simulink model "CaseStudyII_9_Bus"  (R2020a)
settings: Solver=FixedStepAuto  StartTime=0.0  StopTime=Tend  FixedStep=T_s_power  MaxStep=5.0E-5  RelTol=1e-3
values from neighbouring files (symbols this model uses):
  B_s46 = b_s46*Cb    (= 9.5071761847e-07)    [Data_CaseStudyI.m]    (also in Data_CaseStudyII.m; Data_InitialSystem.m)
  B_s54 = b_s54*Cb    (= 1.05902722057e-06)    [Data_CaseStudyI.m]    (also in Data_CaseStudyII.m; Data_InitialSystem.m)
  B_s69 = b_s69*Cb    (= 2.15415764185e-06)    [Data_CaseStudyI.m]    (also in Data_CaseStudyII.m; Data_InitialSystem.m)
  B_s75 = b_s75*Cb    (= 1.84126323577e-06)    [Data_CaseStudyI.m]    (also in Data_CaseStudyII.m; Data_InitialSystem.m)
  B_s87 = b_s87*Cb    (= 8.96562817417e-07)    [Data_CaseStudyI.m]    (also in Data_CaseStudyII.m; Data_InitialSystem.m)
  B_s98 = b_s98*Cb    (= 1.25759482443e-06)    [Data_CaseStudyI.m]    (also in Data_CaseStudyII.m; Data_InitialSystem.m)
  C_dc_DVPP_1_2 = 0.008*(n_DVPP_1_2)    (= 0.8)    [Data_CaseStudyI.m]    (also in Data_CaseStudyII.m)
  C_dc_DVPP_1_3 = 0.008*(n_DVPP_1_3)    (= 0.4)    [Data_CaseStudyI.m]    (also in Data_CaseStudyII.m)
  C_dc_DVPP_3_1 = 0.008*(n_DVPP_3_1)    (= 1.128)    [Data_CaseStudyII.m]
  C_dc_DVPP_3_2 = 0.008*(n_DVPP_3_2)    (= 0.848)    [Data_CaseStudyII.m]
  C_dc_DVPP_3_3 = 0.008*(n_DVPP_3_3)    (= 1.28)    [Data_CaseStudyII.m]
  Dp_DVPP_3_pu = 1/dp_DVPP_3    (= 33.3333333333)    [Data_CaseStudyII.m]
  Dq1_DVPP_3_pu = 100    [Data_CaseStudyII.m]
  fb = 50    [Data_CaseStudyI.m]    (also in Data_CaseStudyII.m; Data_InitialSystem.m)
  HGov_dyn = HGov_delay*H_tr_droop    [Data_CaseStudyI.m]    (also in Data_CaseStudyII.m; Data_InitialSystem.m)
  HTurb_tot = H_water_way    [Data_CaseStudyI.m]    (also in Data_CaseStudyII.m; Data_InitialSystem.m)
  I_m_DVPP_1_2 = 2/3*Sb_DVPP_1_2/V_m_DVPP_1_2    [Data_CaseStudyI.m]    (also in Data_CaseStudyII.m)
  I_m_DVPP_1_3 = 2/3*Sb_DVPP_1_3/V_m_DVPP_1_3    [Data_CaseStudyI.m]    (also in Data_CaseStudyII.m)
  I_m_DVPP_3_1 = 2/3*Sb_DVPP_3_1/V_m_DVPP_3_1    [Data_CaseStudyII.m]
  I_m_DVPP_3_2 = 2/3*Sb_DVPP_3_2/V_m_DVPP_3_2    [Data_CaseStudyII.m]
  I_m_DVPP_3_3 = 2/3*Sb_DVPP_3_3/V_m_DVPP_3_3    [Data_CaseStudyII.m]
  i_star_max = 1.3    [Data_CaseStudyI.m]    (also in Data_CaseStudyII.m)
  iabc_DVPP_1_2_0 = T0*idq0_DVPP_1_2    [Data_CaseStudyI.m]    (also in Data_CaseStudyII.m)
  iabc_DVPP_1_3_0 = T0*idq0_DVPP_1_3    [Data_CaseStudyI.m]    (also in Data_CaseStudyII.m)
  iabc_DVPP_3_1_0 = T0*idq0_DVPP_3_1    [Data_CaseStudyII.m]
  iabc_DVPP_3_2_0 = T0*idq0_DVPP_3_2    [Data_CaseStudyII.m]
  iabc_DVPP_3_3_0 = T0*idq0_DVPP_3_3    [Data_CaseStudyII.m]
  K2_DVPP_1 = [-0.0221795494247 -1.60799665656 0.160449825826 -2.94803557381 -11.8081988371 -9.75170960256 0.00463021906909 -49.1667298155]    [ControlGains_DVPP1.mat]
  K3_DVPP_1 = [-0.0591512752956 -1.61493903379 -27.2946107927 -16.2119211358 -14.3657419818 2.05688388773 -2.27328406162 0.146700393037 -150.920793597]    [ControlGains_DVPP1.mat]
  k_dc_DVPP_1_2 = eta_DVPP_1_2/(Vdc_n_DVPP_1_2*m_p_DVPP_1_2)    [Data_CaseStudyI.m]    (also in Data_CaseStudyII.m)
  k_dc_DVPP_1_3 = eta_DVPP_1_3/(Vdc_n_DVPP_1_3*m_p_DVPP_1_3)    [Data_CaseStudyI.m]    (also in Data_CaseStudyII.m)
  k_dc_DVPP_3_1 = eta_DVPP_3_1/(Vdc_n_DVPP_3_1*m_p_DVPP_3_1)    [Data_CaseStudyII.m]
  k_dc_DVPP_3_2 = eta_DVPP_3_2/(Vdc_n_DVPP_3_2*m_p_DVPP_3_2)    [Data_CaseStudyII.m]
  k_dc_DVPP_3_3 = eta_DVPP_3_3/(Vdc_n_DVPP_3_3*m_p_DVPP_3_3)    [Data_CaseStudyII.m]
  ki_i_pu = 1.19    [Data_CaseStudyI.m]    (also in Data_CaseStudyII.m)
  ki_pll = 1700    [Data_CaseStudyI.m]    (also in Data_CaseStudyII.m)
  ki_q_pu = 0.005    [Data_CaseStudyI.m]    (also in Data_CaseStudyII.m)
  kp_i_pu = 0.73    [Data_CaseStudyI.m]    (also in Data_CaseStudyII.m)
  kp_pll = 150    [Data_CaseStudyI.m]    (also in Data_CaseStudyII.m)
  kp_q_pu = 0.05    [Data_CaseStudyI.m]    (also in Data_CaseStudyII.m)
  L1_DVPP_1_2_pu = 0.0186/m_DVPP_1_2    (= 0.000372)    [Data_CaseStudyI.m]    (also in Data_CaseStudyII.m)
  L1_DVPP_1_3_pu = 0.0186/m_DVPP_1_3    (= 0.000744)    [Data_CaseStudyI.m]    (also in Data_CaseStudyII.m)
  L1_DVPP_3_1_pu = 0.0186/m_DVPP_3_1    (= 0.000263829787234)    [Data_CaseStudyII.m]
  L1_DVPP_3_2_pu = 0.0186/m_DVPP_3_2    (= 0.000350943396226)    [Data_CaseStudyII.m]
  L1_DVPP_3_3_pu = 0.0186/m_DVPP_3_3    (= 0.0002325)    [Data_CaseStudyII.m]
  l1_MVHV1 = 0    [Data_CaseStudyI.m]    (also in Data_CaseStudyII.m; Data_InitialSystem.m)
  l1_MVHV2 = 0    [Data_CaseStudyI.m]    (also in Data_CaseStudyII.m; Data_InitialSystem.m)
  l1_MVHV3 = 0    [Data_CaseStudyI.m]    (also in Data_CaseStudyII.m; Data_InitialSystem.m)
  L2_DVPP_1_2_pu = L1_DVPP_1_2_pu    (= 0.000372)    [Data_CaseStudyI.m]    (also in Data_CaseStudyII.m)
  L2_DVPP_1_3_pu = L1_DVPP_1_3_pu    (= 0.000744)    [Data_CaseStudyI.m]    (also in Data_CaseStudyII.m)
  L2_DVPP_3_1_pu = L1_DVPP_3_1_pu    (= 0.000263829787234)    [Data_CaseStudyII.m]
  L2_DVPP_3_2_pu = L1_DVPP_3_2_pu    (= 0.000350943396226)    [Data_CaseStudyII.m]
  L2_DVPP_3_3_pu = L1_DVPP_3_3_pu    (= 0.0002325)    [Data_CaseStudyII.m]
  l2_MVHV1 = l_s14    (= 0.0576)    [Data_CaseStudyI.m]    (also in Data_CaseStudyII.m; Data_InitialSystem.m)
  l2_MVHV2 = l_s72    (= 0.0625)    [Data_CaseStudyI.m]    (also in Data_CaseStudyII.m; Data_InitialSystem.m)
  l2_MVHV3 = l_s39    (= 0.0586)    [Data_CaseStudyI.m]    (also in Data_CaseStudyII.m; Data_InitialSystem.m)
  l_f_DVPP_1_2 = L_f_DVPP_1_2*w_b/Zb_DVPP_1_2    [Data_CaseStudyI.m]    (also in Data_CaseStudyII.m)
  L_f_DVPP_1_2 = (1/(n_DVPP_1_2))*600*10^-6    (= 6e-06)    [Data_CaseStudyI.m]    (also in Data_CaseStudyII.m)
  l_f_DVPP_1_3 = L_f_DVPP_1_3*w_b/Zb_DVPP_1_3    [Data_CaseStudyI.m]    (also in Data_CaseStudyII.m)
  L_f_DVPP_1_3 = (1/(n_DVPP_1_3))*600*10^-6    (= 1.2e-05)    [Data_CaseStudyI.m]    (also in Data_CaseStudyII.m)
  l_f_DVPP_3_1 = L_f_DVPP_3_1*w_b/Zb_DVPP_3_1    [Data_CaseStudyII.m]
  L_f_DVPP_3_1 = (1/(n_DVPP_3_1))*600*10^-6    (= 4.25531914894e-06)    [Data_CaseStudyII.m]
  l_f_DVPP_3_2 = L_f_DVPP_3_2*w_b/Zb_DVPP_3_2    [Data_CaseStudyII.m]
  L_f_DVPP_3_2 = (1/(n_DVPP_3_2))*600*10^-6    (= 5.66037735849e-06)    [Data_CaseStudyII.m]
  l_f_DVPP_3_3 = L_f_DVPP_3_3*w_b/Zb_DVPP_3_3    [Data_CaseStudyII.m]
  L_f_DVPP_3_3 = (1/(n_DVPP_3_3))*600*10^-6    (= 3.75e-06)    [Data_CaseStudyII.m]
  L_s46 = l_s46*Lb    (= 0.154915055408)    [Data_CaseStudyI.m]    (also in Data_CaseStudyII.m; Data_InitialSystem.m)
  L_s54 = l_s54*Lb    (= 0.143128040323)    [Data_CaseStudyI.m]    (also in Data_CaseStudyII.m; Data_InitialSystem.m)
  L_s69 = l_s69*Lb    (= 0.286256080645)    [Data_CaseStudyI.m]    (also in Data_CaseStudyII.m; Data_InitialSystem.m)
  L_s75 = l_s75*Lb    (= 0.271101346964)    [Data_CaseStudyI.m]    (also in Data_CaseStudyII.m; Data_InitialSystem.m)
  L_s87 = l_s87*Lb    (= 0.12123786945)    [Data_CaseStudyI.m]    (also in Data_CaseStudyII.m; Data_InitialSystem.m)
  L_s98 = l_s98*Lb    (= 0.16973301723)    [Data_CaseStudyI.m]    (also in Data_CaseStudyII.m; Data_InitialSystem.m)
  LPV_K1_DVPP_3 = [0.014519129833 -1.24253756746e-17 -0.00331576987938 -1.41950397655e-17 -0.00331577010739 -1.6423216922e-19 0.0145191298795 1.47256053017e-18 1.92456501739e-17 0.00968260817745 7.5102914291e-19 0.0096826081765 ... (80 elements, 8x10)]    [ControlGains_DVPP3_LPV.mat]
  LPV_K2_DVPP_3 = [0.0299413265511 -2.72480441208e-16 -0.00563144274341 -6.63344905835e-17 -0.00563144273182 -1.08918556426e-16 0.0299413268326 -1.32404731664e-16 -4.78559537004e-17 -0.00914230292149 -8.50409089014e-21 -0.00914230292147 ... (80 elements, 8x10)]    [ControlGains_DVPP3_LPV.mat]
  LPV_K3_DVPP_3 = [-0.0173301370849 5.00398589077e-17 -0.0636125194304 3.31757376688e-17 -0.0636125164794 5.41726806116e-17 -0.017330137145 2.43427565927e-17 -0.0400570975704 -5.68753124238e-17 -0.0574012283733 2.45717741258e-17 ... (192 elements, 16x12)]    [ControlGains_DVPP3_LPV.mat]
  Mp_DVPP_3_pu = 13    [Data_CaseStudyII.m]
  P_L = pL*Sb    (= 300000000)    [Data_CaseStudyI.m]    (also in Data_CaseStudyII.m; Data_InitialSystem.m)
  p_set_bus1 = P_set_bus1/SbSG1    (= 0.731707317073)    [Data_CaseStudyI.m]    (also in Data_CaseStudyII.m; Data_InitialSystem.m)
  p_set_bus2 = P_set_bus2/SbSG2    (= 0.756707317073)    [Data_CaseStudyI.m]    (also in Data_CaseStudyII.m; Data_InitialSystem.m)
  Pb_DVPP_3_1 = 37e6    (= 37000000)    [Data_CaseStudyII.m]
  Pb_DVPP_3_2 = 28e6    (= 28000000)    [Data_CaseStudyII.m]
  Pb_DVPP_3_3 = 0e6    (= 0)    [Data_CaseStudyII.m]
  pset_DVPP_1_1 = P_set_bus1/SbSG1    (= 0.731707317073)    [Data_CaseStudyI.m]    (also in Data_CaseStudyII.m)
  pset_DVPP_1_2 = 0    [Data_CaseStudyI.m]    (also in Data_CaseStudyII.m)
  pset_DVPP_1_3 = 0    [Data_CaseStudyI.m]    (also in Data_CaseStudyII.m)
  pset_DVPP_3_1 = (0.6*P_set_bus3)/Sb_DVPP_3_1    (= 0.398546964193)    [Data_CaseStudyII.m]
  pset_DVPP_3_2 = (0.4*P_set_bus3)/Sb_DVPP_3_2    (= 0.353428439945)    [Data_CaseStudyII.m]
  pset_DVPP_3_3 = 0    [Data_CaseStudyII.m]
  Q_L = qL*Sb    (= 82500000)    [Data_CaseStudyI.m]    (also in Data_CaseStudyII.m; Data_InitialSystem.m)
  qset_DVPP_1_2 = 0    [Data_CaseStudyI.m]    (also in Data_CaseStudyII.m)
  qset_DVPP_1_3 = 0    [Data_CaseStudyI.m]    (also in Data_CaseStudyII.m)
  qset_DVPP_3_1 = 0    [Data_CaseStudyII.m]
  qset_DVPP_3_2 = 0    [Data_CaseStudyII.m]
  qset_DVPP_3_3 = 0    [Data_CaseStudyII.m]
  R1_DVPP_1_2_pu = 0.00734/m_DVPP_1_2    (= 0.0001468)    [Data_CaseStudyI.m]    (also in Data_CaseStudyII.m)
  R1_DVPP_1_3_pu = 0.00734/m_DVPP_1_3    (= 0.0002936)    [Data_CaseStudyI.m]    (also in Data_CaseStudyII.m)
  R1_DVPP_3_1_pu = 0.00734/m_DVPP_3_1    (= 0.000104113475177)    [Data_CaseStudyII.m]
  R1_DVPP_3_2_pu = 0.00734/m_DVPP_3_2    (= 0.000138490566038)    [Data_CaseStudyII.m]
  R1_DVPP_3_3_pu = 0.00734/m_DVPP_3_3    (= 9.175e-05)    [Data_CaseStudyII.m]
  r1_MVHV1 = 1e-6    (= 1e-06)    [Data_CaseStudyI.m]    (also in Data_CaseStudyII.m; Data_InitialSystem.m)
  r1_MVHV2 = 1e-6    (= 1e-06)    [Data_CaseStudyI.m]    (also in Data_CaseStudyII.m; Data_InitialSystem.m)
  r1_MVHV3 = 1e-6    (= 1e-06)    [Data_CaseStudyI.m]    (also in Data_CaseStudyII.m; Data_InitialSystem.m)
  R2_DVPP_1_2_pu = R1_DVPP_1_2_pu    (= 0.0001468)    [Data_CaseStudyI.m]    (also in Data_CaseStudyII.m)
  R2_DVPP_1_3_pu = R1_DVPP_1_3_pu    (= 0.0002936)    [Data_CaseStudyI.m]    (also in Data_CaseStudyII.m)
  R2_DVPP_3_1_pu = R1_DVPP_3_1_pu    (= 0.000104113475177)    [Data_CaseStudyII.m]
  R2_DVPP_3_2_pu = R1_DVPP_3_2_pu    (= 0.000138490566038)    [Data_CaseStudyII.m]
  R2_DVPP_3_3_pu = R1_DVPP_3_3_pu    (= 9.175e-05)    [Data_CaseStudyII.m]
  r2_MVHV1 = 1e-6    (= 1e-06)    [Data_CaseStudyI.m]    (also in Data_CaseStudyII.m; Data_InitialSystem.m)
  r2_MVHV2 = 1e-6    (= 1e-06)    [Data_CaseStudyI.m]    (also in Data_CaseStudyII.m; Data_InitialSystem.m)
  r2_MVHV3 = 1e-6    (= 1e-06)    [Data_CaseStudyI.m]    (also in Data_CaseStudyII.m; Data_InitialSystem.m)
  R_dc_DVPP_1_2 = (Vdc_n_DVPP_1_2/(0.05*(Sb_DVPP_1_2)/Vdc_n_DVPP_1_2))    [Data_CaseStudyI.m]    (also in Data_CaseStudyII.m)
  R_dc_DVPP_1_3 = (Vdc_n_DVPP_1_3/(0.05*(Sb_DVPP_1_3)/Vdc_n_DVPP_1_3))    [Data_CaseStudyI.m]    (also in Data_CaseStudyII.m)
  R_dc_DVPP_3_1 = (Vdc_n_DVPP_3_1/(0.05*(Sb_DVPP_3_1)/Vdc_n_DVPP_3_1))    [Data_CaseStudyII.m]
  R_dc_DVPP_3_2 = (Vdc_n_DVPP_3_2/(0.05*(Sb_DVPP_3_2)/Vdc_n_DVPP_3_2))    [Data_CaseStudyII.m]
  R_dc_DVPP_3_3 = (Vdc_n_DVPP_3_3/(0.05*(Sb_DVPP_3_3)/Vdc_n_DVPP_3_3))    [Data_CaseStudyII.m]
  r_f_DVPP_1_2 = R_f_DVPP_1_2/Zb_DVPP_1_2    [Data_CaseStudyI.m]    (also in Data_CaseStudyII.m)
  R_f_DVPP_1_2 = 0.02/n_DVPP_1_2    (= 0.0002)    [Data_CaseStudyI.m]    (also in Data_CaseStudyII.m)
  r_f_DVPP_1_3 = R_f_DVPP_1_3/Zb_DVPP_1_3    [Data_CaseStudyI.m]    (also in Data_CaseStudyII.m)
  R_f_DVPP_1_3 = 0.02/n_DVPP_1_3    (= 0.0004)    [Data_CaseStudyI.m]    (also in Data_CaseStudyII.m)
  r_f_DVPP_3_1 = R_f_DVPP_3_1/Zb_DVPP_3_1    [Data_CaseStudyII.m]
  ... (+104 more)
undefined symbols (not defined in the file or in its folder): A, B, C, Continuous, Dd, Efd0, gcbh, i_dc, Ka, Kf, p2set, SbSM2, sps_rtmsupport, spsST1AModel, Ta, Tb, Tb1, Tc, Tc1, Tf, VA0, VAmax, VAmin, VImax, VImin, VRmax, VRmin
libraries: powerlib x95, powerlib_meascontrol x41, cstblocks x15, sps_avr x1, simulink_extras x1, simulink x1
(part 3 of 5)

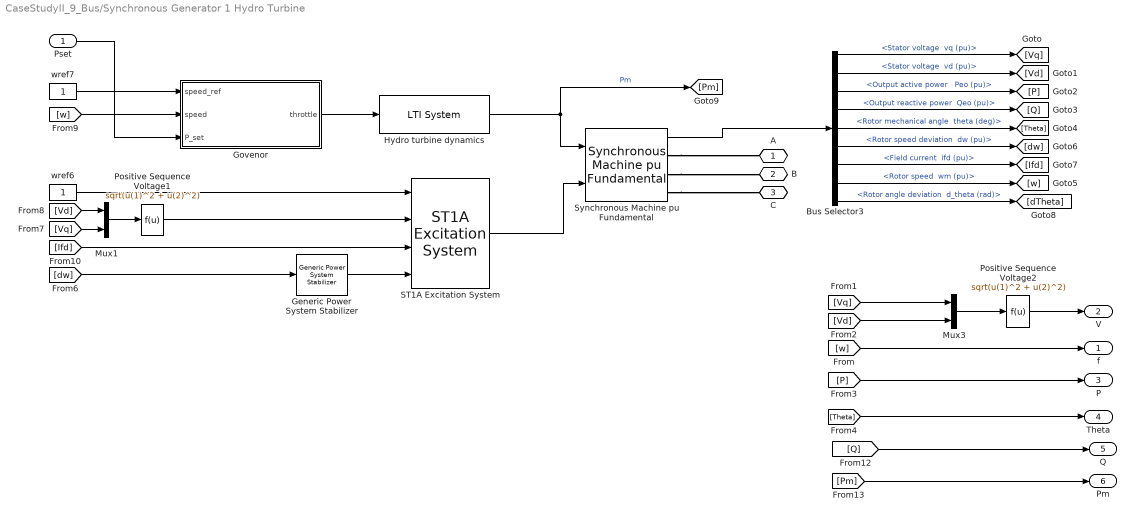
== system CaseStudyII_9_Bus/Synchronous Generator 1 Hydro Turbine ==
  Pset : Inport
  Bus Selector3 : BusSelector  OutputSignals="dq0 components.Stator voltage  vq (pu),dq0 components.Stator voltage  vd (pu),Output active power   Peo (pu),Output reactive power  Qeo (pu),Mechanical.Rotor mechanical angle  theta (deg),Mechanical.Rotor speed deviation  dw (pu),dq0 components.Field current  ifd (pu),Mechanical.Rotor speed  wm (pu),Mechanical.Rotor angle deviation  d_theta (rad)"
  Generic Power System Stabilizer : powerlib/Machines/Generic Power System Stabilizer  Tsensor=30e-3  K=15  Twashout=1  Tleadlag1=[50e-3 20e-3]  Tleadlag2=[3 5.4]  VSlimits=[-0.15 0.15]  Vinit=0  Plot_On=off  MagdB_On=on  FreqRange=logspace(-2,2,500)
      settings: SourceProductBaseCode=PS
  Govenor : Subsystem
  Hydro turbine dynamics : cstblocks/LTI System  sys=ss(HTurb_tot)  IC=p_set_bus1/3
  Mux1 : Mux  Inputs=2
  Mux3 : Mux  Inputs=2
  Positive Sequence Voltage1 : Fcn  Expr=sqrt(u(1)^2 + u(2)^2)
  Positive Sequence Voltage2 : Fcn  Expr=sqrt(u(1)^2 + u(2)^2)
  ST1A Excitation System : sps_avr/ST1A Excitation System  Tr=20e-3  KaTa=[210 0.001]  VIminmax=[-999 +999]  VAminmax=[-999 999]  VRminmax=[-6.0 6.43]  KfTf=[0.001 1]  TbTc=[0 0 0 0]  KLR=1  ILR=2  Kc=0.038  v0=[1 1.7165]  TsBlock=0
      settings: SourceProductBaseCode=PS
  Synchronous Machine pu Fundamental : powerlib/Machines/Synchronous Machine pu Fundamental  PresetModel=No  MechanicalLoad=Mechanical power Pm  ShowDetailedParameters=on  RotorType=Round  Units=per unit fundamental parameters  MeasurementBus=off  NominalParameters="[SbSG1  VbMV1   fb]"  Stator="[ 2.85E-03  0.114  1.19  0.36 ]"  Field="[ 5.79E-04  0.114]"  Dampers2=[0.0652, 0.5134, 0.0287, 0.2553, 7.765e-3, 0.9167 ]  Dampers1="[ 1.17E-02  0.182  1.97E-02  0.384 ]"  Mechanical=[6 0.0032 20]  PolePairs=20  InitialConditions=[0 0 0 0 0 0 0 0 1]  SetSaturation=off  Saturation=[0.6404,0.7127,0.8441,0.9214,0.9956,1.082,1.19,1.316,1.457;0.7,0.7698,0.8872,0.9466,0.9969,1.046,1.1,1.151,1.201]  LoadFlowParameters=[1,0,0,0,0]  TsPowergui=0  TsBlock=-1  IterativeModel=Trapezoidal non iterative  IterativeDiscreteModel=Trapezoidal non iterative  BusType=swing  Pref=p2set*SbSM2  Qref=0  Qmin=-inf  Qmax=inf  PLF=0  QLF=0
      settings: SourceProductBaseCode=PS
  wref6 : Constant
  wref7 : Constant
  A : PMIOPort  Side=Right
  B : PMIOPort  Port=2  Side=Right
  C : PMIOPort  Port=3  Side=Right
  f : Outport  VectorParamsAs1DForOutWhenUnconnected=off
  V : Outport  Port=2  VectorParamsAs1DForOutWhenUnconnected=off
  P : Outport  Port=3  VectorParamsAs1DForOutWhenUnconnected=off
  Theta : Outport  Port=4  VectorParamsAs1DForOutWhenUnconnected=off
  Q : Outport  Port=5  VectorParamsAs1DForOutWhenUnconnected=off
  Pm : Outport  Port=6  VectorParamsAs1DForOutWhenUnconnected=off
  wires:
  ST1A Excitation System/1 -> Synchronous Machine pu Fundamental/2
  [dw] -> Generic Power System Stabilizer/1
  Bus Selector3/8 -> [w]  "<Rotor speed  wm (pu)>"
  Bus Selector3/7 -> [Ifd]  "<Field current  ifd (pu)>"
  Bus Selector3/6 -> [dw]  "<Rotor speed deviation  dw (pu)>"
  Bus Selector3/5 -> [Theta]  "<Rotor mechanical angle  theta (deg)>"
  Bus Selector3/4 -> [Q]  "<Output reactive power  Qeo (pu)>"
  Bus Selector3/3 -> [P]  "<Output active power   Peo (pu)>"
  Bus Selector3/2 -> [Vd]  "<Stator voltage  vd (pu)>"
  Bus Selector3/1 -> [Vq]  "<Stator voltage  vq (pu)>"
  [Theta] -> Theta/1
  [P] -> P/1
  [Vd] -> Mux3/2
  [Vq] -> Mux3/1
  Synchronous Machine pu Fundamental/1 -> Bus Selector3/1
  Mux3/1 -> Positive Sequence Voltage2/1
  wref6/1 -> ST1A Excitation System/1
  Positive Sequence Voltage2/1 -> V/1
  [w] -> f/1
  Bus Selector3/9 -> [dTheta]  "<Rotor angle deviation  d_theta (rad)>"
  Mux1/1 -> Positive Sequence Voltage1/1
  [Vd] -> Mux1/1
  [Vq] -> Mux1/2
  Generic Power System Stabilizer/1 -> ST1A Excitation System/4
  Govenor/1(throttle) -> Hydro turbine dynamics/1
  [Q] -> Q/1
  Positive Sequence Voltage1/1 -> ST1A Excitation System/2
  [Ifd] -> ST1A Excitation System/3
  wref7/1 -> Govenor/1(speed_ref)
  Pset/1 -> Govenor/3(P_set)
  [Pm] -> Pm/1
  [w] -> Govenor/2(speed)
  Hydro turbine dynamics/1 -> Synchronous Machine pu Fundamental/1, [Pm]  "Pm"
  connections:
  Synchronous Machine pu Fundamental/RConn2 -- B/RConn1
  Synchronous Machine pu Fundamental/RConn3 -- C/RConn1
  Synchronous Machine pu Fundamental/RConn1 -- A/RConn1

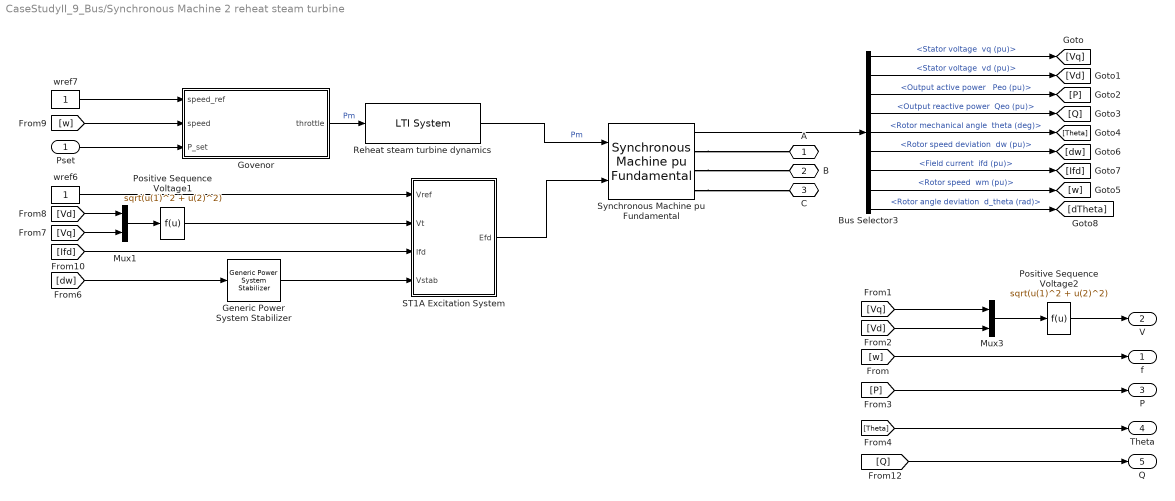
== system CaseStudyII_9_Bus/Synchronous Machine 2 reheat steam turbine ==
  Pset : Inport
  Bus Selector3 : BusSelector  OutputSignals="dq0 components.Stator voltage  vq (pu),dq0 components.Stator voltage  vd (pu),Output active power   Peo (pu),Output reactive power  Qeo (pu),Mechanical.Rotor mechanical angle  theta (deg),Mechanical.Rotor speed deviation  dw (pu),dq0 components.Field current  ifd (pu),Mechanical.Rotor speed  wm (pu),Mechanical.Rotor angle deviation  d_theta (rad)"
  Generic Power System Stabilizer : powerlib/Machines/Generic Power System Stabilizer  Tsensor=30e-3  K=15  Twashout=1  Tleadlag1=[50e-3 20e-3]  Tleadlag2=[3 5.4]  VSlimits=[-0.15 0.15]  Vinit=0  Plot_On=off  MagdB_On=on  FreqRange=logspace(-2,2,500)
      settings: SourceProductBaseCode=PS
  Govenor : Subsystem
  Mux1 : Mux  Inputs=2
  Mux3 : Mux  Inputs=2
  Positive Sequence Voltage1 : Fcn  Expr=sqrt(u(1)^2 + u(2)^2)
  Positive Sequence Voltage2 : Fcn  Expr=sqrt(u(1)^2 + u(2)^2)
  Reheat steam turbine dynamics : cstblocks/LTI System  sys=ss(STurb_reheat)  IC=[1 0.2281]
  ST1A Excitation System : Subsystem  AncestorBlock=sps_avr/ST1A Excitation System  DialogController=POWERSYS.PowerSysDialog  LoadFcn=sps_rtmsupport('LoadFcn', gcbh);  StartFcn=sps_rtmsupport('StartFcn', gcbh);  StopFcn=sps_rtmsupport('StopFcn', gcbh);  mask(ST1A Excitation System){Tr=20e-3, KaTa=[210 0.001], VIminmax=[-999 +999], VAminmax=[-999 999], VRminmax=[-6.0 6.43], KfTf=[0.001 1], TbTc=[0 0 0 0], KLR=1, ILR=2, Kc=0.038, v0=[1 1.6825], TsBlock=0}
      mask prompts: Tr "Low-pass filter time constant Tr(s):"; KaTa "Voltage regulator gain and time constant [Ka Ta(s)]:"; VIminmax "Voltage regulator input limits [VImin(pu) VImax(pu)]:"; VAminmax "Voltage regulator internal limits [VAmin(pu) VAmax(pu)]:"; VRminmax "Voltage regulator output limits [VRmin(pu) VRmax(pu)]:"; KfTf "Damping filter gain and time constant [Kf Tf(s)]:"; TbTc "Transient gain reduction lead and lag time constants [Tb(s) Tc(s) Tb1(s) Tc1(s)]:"; KLR "Exciter output current limiter gain KLR(pu):"; ILR "Exciter output current limit reference ILR(pu):"; Kc "Rectifier loading factor Kc(pu):"; v0 "Initial values of terminal voltage and field voltage [Vt0(pu) Efd0(pu)]:"; TsBlock "Sample time:"
      mask help: Implements a synchronous machine voltage regulator and exciter based on the IEEE type ST1A excitation system model. The output is the field voltage to apply to the Vf input of a Synchronous Machine block. Inputs and output are in p.u.
      mask init:
      | block = gcb;
      | [Ts,BlockChoice,MaskType,Ka,Ta,Kf,Tf,Tb,Tc,Tb1,Tc1,VRmin,VRmax,VImin,VImax,VAmin,VAmax,Ifd0,VA0,Vt0,Efd0] = powericon('ExcitationSystemInit',block,TsBlock,KaTa,KfTf,TbTc,VRminmax,VIminmax,VAminmax,Kc,ILR,KLR,v0);
      | powericon('SetInternalModels','set',block,BlockChoice);
      settings: CopyFcn=sps_rtmsupport('CopyFcn', gcbh);  DeleteFcn=sps_rtmsupport('DeleteFcn', gcbh);  UndoDeleteFcn=sps_rtmsupport('UndoDeleteFcn', gcbh);  ModelCloseFcn=sps_rtmsupport('ModelCloseFcn', gcbh);  PreSaveFcn=sps_rtmsupport('PreSaveFcn', gcbh);  PostSaveFcn=sps_rtmsupport('PostSaveFcn', gcbh);  NameChangeFcn=sps_rtmsupport('NameChangeFcn', gcbh);  PreCopyFcn=sps_rtmsupport('PreCopyFcn', gcbh);  OpenFcn=sps_rtmsupport('OpenFcn', gcbh, []);  CloseFcn=sps_rtmsupport('CloseFcn', gcbh);  PreDeleteFcn=sps_rtmsupport('PreDeleteFcn', gcbh);
      mask Help: helpview(psbhelp);
      mask Display: color('blue');disp('ST1A')
  Synchronous Machine pu Fundamental : powerlib/Machines/Synchronous Machine pu Fundamental  PresetModel=No  MechanicalLoad=Mechanical power Pm  ShowDetailedParameters=on  RotorType=Round  Units=per unit fundamental parameters  MeasurementBus=off  NominalParameters="[ SbSG2  VbMV2   fb]"  Stator="[ 2.85E-03  0.114  1.19  0.36 ]"  Field="[ 5.79E-04  0.114]"  Dampers2=[0.0652, 0.5134, 0.0287, 0.2553, 7.765e-3, 0.9167 ]  Dampers1="[ 1.17E-02  0.182  1.97E-02  0.384 ]"  Mechanical=[13 0 20]  PolePairs=20  InitialConditions=[0 0 0 0 0 0 0 0 1]  SetSaturation=off  Saturation=[0.6404,0.7127,0.8441,0.9214,0.9956,1.082,1.19,1.316,1.457;0.7,0.7698,0.8872,0.9466,0.9969,1.046,1.1,1.151,1.201]  LoadFlowParameters=[1,0,0,0,0]  TsPowergui=0  TsBlock=-1  IterativeModel=Trapezoidal non iterative  IterativeDiscreteModel=Trapezoidal non iterative  BusType=PV  Pref=P_set_bus2  Qref=0  Qmin=-inf  Qmax=inf  PLF=0  QLF=0
      settings: SourceProductBaseCode=PS
  wref6 : Constant
  wref7 : Constant
  A : PMIOPort  Side=Right
  B : PMIOPort  Port=2  Side=Right
  C : PMIOPort  Port=3  Side=Right
  f : Outport  VectorParamsAs1DForOutWhenUnconnected=off
  V : Outport  Port=2  VectorParamsAs1DForOutWhenUnconnected=off
  P : Outport  Port=3  VectorParamsAs1DForOutWhenUnconnected=off
  Theta : Outport  Port=4  VectorParamsAs1DForOutWhenUnconnected=off
  Q : Outport  Port=5  VectorParamsAs1DForOutWhenUnconnected=off
  wires:
  ST1A Excitation System/1(Efd) -> Synchronous Machine pu Fundamental/2
  [dw] -> Generic Power System Stabilizer/1
  Generic Power System Stabilizer/1 -> ST1A Excitation System/4(Vstab)
  Bus Selector3/8 -> [w]  "<Rotor speed  wm (pu)>"
  Bus Selector3/7 -> [Ifd]  "<Field current  ifd (pu)>"
  Bus Selector3/6 -> [dw]  "<Rotor speed deviation  dw (pu)>"
  Bus Selector3/5 -> [Theta]  "<Rotor mechanical angle  theta (deg)>"
  Bus Selector3/4 -> [Q]  "<Output reactive power  Qeo (pu)>"
  Bus Selector3/3 -> [P]  "<Output active power   Peo (pu)>"
  Bus Selector3/2 -> [Vd]  "<Stator voltage  vd (pu)>"
  Bus Selector3/1 -> [Vq]  "<Stator voltage  vq (pu)>"
  [Theta] -> Theta/1
  [P] -> P/1
  [Vd] -> Mux3/2
  [Vq] -> Mux3/1
  Synchronous Machine pu Fundamental/1 -> Bus Selector3/1
  Mux3/1 -> Positive Sequence Voltage2/1
  wref6/1 -> ST1A Excitation System/1(Vref)
  Positive Sequence Voltage2/1 -> V/1
  [w] -> f/1
  Bus Selector3/9 -> [dTheta]  "<Rotor angle deviation  d_theta (rad)>"
  Mux1/1 -> Positive Sequence Voltage1/1
  [Vd] -> Mux1/1
  [Vq] -> Mux1/2
  [w] -> Govenor/2(speed)
  wref7/1 -> Govenor/1(speed_ref)
  [Q] -> Q/1
  Govenor/1(throttle) -> Reheat steam turbine dynamics/1  "Pm"
  Positive Sequence Voltage1/1 -> ST1A Excitation System/2(Vt)
  [Ifd] -> ST1A Excitation System/3(Ifd)
  Pset/1 -> Govenor/3(P_set)
  Reheat steam turbine dynamics/1 -> Synchronous Machine pu Fundamental/1  "Pm"
  connections:
  Synchronous Machine pu Fundamental/RConn2 -- B/RConn1
  Synchronous Machine pu Fundamental/RConn3 -- C/RConn1
  Synchronous Machine pu Fundamental/RConn1 -- A/RConn1

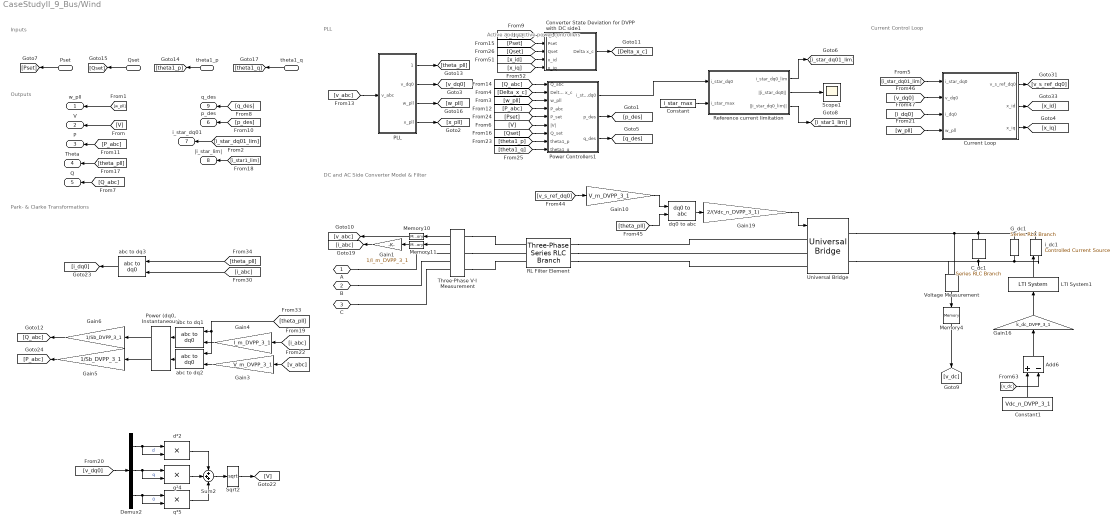
== system CaseStudyII_9_Bus/Wind  ==
  note: Current Control Loop
  note: Outputs
  note: Inputs
  note: PLL
  note: Park- & Clarke Transformations
  note: Active and reactive power controllers
  note: DC and AC Side Converter Model & Filter
  Pset : Inport
  Qset : Inport  Port=2
  theta1_p : Inport  Port=3
  theta1_q : Inport  Port=4
  Add6 : Sum  Inputs=+-
  C_dc1 : powerlib/Elements/Series RLC Branch  LConnTagsString=__new0  RConnTagsString=__new0  BranchType=C  Resistance=1  Inductance=1e-3  SetiL0=off  InitialCurrent=0  Capacitance=C_dc_DVPP_3_1  Setx0=off  InitialVoltage=Vdc_n  Measurements=None
  Constant : Constant  Value=i_star_max
  Constant1 : Constant  Value=Vdc_n_DVPP_3_1
  Converter State Deviation for DVPP with DC side1 : Subsystem
  Current Loop : Subsystem  AncestorBlock=Library/Grid-Forming Converter Controlled by Droop Control /Current Loop
  Demux2 : Demux  Outputs=3
  G_dc1 : powerlib/Elements/Series RLC Branch  LConnTagsString=__new0  RConnTagsString=__new0  BranchType=R  Resistance=R_dc_DVPP_3_1  Inductance=1e-3  SetiL0=off  InitialCurrent=0  Capacitance=1e-6  Setx0=off  InitialVoltage=0  Measurements=None
  Gain1 : Gain  Gain=1/I_m_DVPP_3_1
  Gain10 : Gain  Gain=V_m_DVPP_3_1
  Gain16 : Gain  Gain=k_dc_DVPP_3_1
  Gain19 : Gain  Gain=2/(Vdc_n_DVPP_3_1)
  Gain3 : Gain  Gain=V_m_DVPP_3_1
  Gain4 : Gain  Gain=I_m_DVPP_3_1
  Gain5 : Gain  Gain=1/Sb_DVPP_3_1
  Gain6 : Gain  Gain=1/Sb_DVPP_3_1
  LTI System1 : cstblocks/LTI System  sys=tf(1,[tau_dc_DVPP_3_1 1])  IC=[]
  Memory10 : Memory  InitialCondition=[vabc_DVPP_3_1_0_pu(1), vabc_DVPP_3_1_0_pu(2), vabc_DVPP_3_1_0_pu(3)]
  Memory11 : Memory  InitialCondition=[iabc_DVPP_3_1_0(1), iabc_DVPP_3_1_0(2), iabc_DVPP_3_1_0(3)]
  Memory4 : Memory
  PLL : Subsystem
  "Power (dq0, Instantaneous)" : powerlib_meascontrol/Measurements/Power (dq0, Instantaneous)
      settings: SourceProductBaseCode=PS
  Power Controllers1 : Subsystem
  RL Filter Element : powerlib/Elements/Three-Phase Series RLC Branch  LConnTagsString=A|B|C  RConnTagsString=A|B|C  BranchType=RL  Resistance=R_f_DVPP_3_1  Inductance=L_f_DVPP_3_1  Capacitance=0  Measurements=Branch currents
  Reference current limitation : Subsystem
  Scope1 : Scope
  Sqrt2 : Sqrt  SaturateOnIntegerOverflow=on
  Sum2 : Sum  Inputs=+++  InputSameDT=on  SaturateOnIntegerOverflow=on  OutDataTypeStr=Inherit: Same as first input
  Three-Phase V-I Measurement : powerlib/Measurements/Three-Phase V-I Measurement  VoltageMeasurement=phase-to-ground  SetLabelV=off  LabelV=Vabc  Vpu=on  VpuLL=off  CurrentMeasurement=yes  SetLabelI=off  LabelI=Iabc  Ipu=off  Pbase=Sb_conv  Vbase=VbLV_DVPP_3_1  OutputType=Complex  PhasorSimulation=off  PSBequivalent=0
  Universal Bridge : powerlib/Power Electronics/Universal Bridge  Arms=3  SnubberResistance=1e5  SnubberCapacitance=inf  Device=Average-model based VSC  Ron=1e-3  Lon=0  ForwardVoltages="[  0  0  ]"  ForwardVoltage=0  GTOparameters=[ 10e-6 , 20e-6 ]  IGBTparameters=[ 1e-6 , 2e-6 ]  Measurements=None  Measurements_2=None  converterType=Rectifier
  Voltage Measurement : powerlib/Measurements/Voltage Measurement  PhasorSimulation=off  OutputType=Complex  PSBequivalent=0
  abc to dq1 : powerlib_meascontrol/Transformations/abc to dq0  Alignment=90 degrees behind phase A axis
  abc to dq2 : powerlib_meascontrol/Transformations/abc to dq0  Alignment=90 degrees behind phase A axis
  abc to dq3 : powerlib_meascontrol/Transformations/abc to dq0  Alignment=90 degrees behind phase A axis
  dq0 to abc : powerlib_meascontrol/Transformations/dq0 to abc  Alignment=90 degrees behind phase A axis
  d²2 : Product  InputSameDT=on  RndMeth=Zero  SaturateOnIntegerOverflow=on  OutDataTypeStr=Inherit: Same as first input
  i_dc1 : powerlib/Electrical Sources/Controlled Current Source  Initialize=off  Source_Type=DC  Amplitude=i_dc  Phase=0  Frequency=0  Measurements=None
  q²4 : Product  InputSameDT=on  RndMeth=Zero  SaturateOnIntegerOverflow=on  OutDataTypeStr=Inherit: Same as first input
  q²5 : Product  InputSameDT=on  RndMeth=Zero  SaturateOnIntegerOverflow=on  OutDataTypeStr=Inherit: Same as first input
  A : PMIOPort  Side=Right
  B : PMIOPort  Port=2  Side=Right
  C : PMIOPort  Port=3  Side=Right
  w_pll : Outport  VectorParamsAs1DForOutWhenUnconnected=off
  V : Outport  Port=2  VectorParamsAs1DForOutWhenUnconnected=off
  P : Outport  Port=3  VectorParamsAs1DForOutWhenUnconnected=off
  Theta : Outport  Port=4  VectorParamsAs1DForOutWhenUnconnected=off
  Q : Outport  Port=5  VectorParamsAs1DForOutWhenUnconnected=off
  p_des : Outport  Port=6  VectorParamsAs1DForOutWhenUnconnected=off
  i_star_dq01 : Outport  Port=7  VectorParamsAs1DForOutWhenUnconnected=off
  |i_star_lim| : Outport  Port=8  VectorParamsAs1DForOutWhenUnconnected=off
  q_des : Outport  Port=9  VectorParamsAs1DForOutWhenUnconnected=off
  wires:
  Memory11/1 -> Gain1/1
  [theta_pll] -> Theta/1
  [P_abc] -> P/1
  Voltage Measurement/1 -> Memory4/1
  Three-Phase V-I Measurement/1 -> Memory10/1
  [v_dq0] -> Demux2/1
  Reference current limitation/3(||i_star_dq0_lim||) -> [i_star1_lim]
  [v_s_ref_dq0] -> Gain10/1
  Memory4/1 -> [v_dc]
  Current Loop/1(v_s_ref_dq0) -> [v_s_ref_dq0]
  Constant1/1 -> Add6/1
  abc to dq3/1 -> [i_dq0]
  [theta_pll] -> abc to dq3/2
  Demux2/2 -> q²4/1, q²4/2  "q"
  [w_pll] -> Current Loop/4(w_pll)
  Reference current limitation/1(i_star_dq0_lim) -> [i_star_dq01_lim]
  Gain16/1 -> LTI System1/1
  [theta_pll] -> dq0 to abc/2
  Gain19/1 -> Universal Bridge/1
  [v_abc] -> PLL/1(v_abc)
  [theta_pll] -> abc to dq2/2, abc to dq1/2
  Sqrt2/1 -> [V]
  "Power (dq0, Instantaneous)"/1 -> Gain5/1
  [i_abc] -> abc to dq3/1
  abc to dq2/1 -> "Power (dq0, Instantaneous)"/1
  [Q_abc] -> Q/1
  "Power (dq0, Instantaneous)"/2 -> Gain6/1
  [v_dc] -> Add6/2
  q²5/1 -> Sum2/3
  Add6/1 -> Gain16/1
  dq0 to abc/1 -> Gain19/1
  [i_star1_lim] -> |i_star_lim|/1
  Demux2/3 -> q²5/2, q²5/1  "0"
  Gain6/1 -> [Q_abc]
  Gain5/1 -> [P_abc]
  Sum2/1 -> Sqrt2/1
  Gain10/1 -> dq0 to abc/1
  [i_star_dq01_lim] -> i_star_dq01/1
  d²2/1 -> Sum2/1
  PLL/1(theta_pll) -> [theta_pll]
  [i_dq0] -> Current Loop/3(i_dq0)
  Gain1/1 -> [i_abc]
  [i_abc] -> Gain4/1
  [v_abc] -> Gain3/1
  [w_pll] -> w_pll/1
  Current Loop/2(x_id) -> [x_id]
  [V] -> V/1
  [v_dq0] -> Current Loop/2(v_dq0)
  Pset/1 -> [Pset]
  Qset/1 -> [Qset]
  Three-Phase V-I Measurement/2 -> Memory11/1
  Constant/1 -> Reference current limitation/2(i_star_max)
  abc to dq1/1 -> "Power (dq0, Instantaneous)"/2
  Gain3/1 -> abc to dq2/1
  PLL/3(w_pll) -> [w_pll]
  Reference current limitation/2(||i_star_dq0||) -> Scope1/1
  Demux2/1 -> d²2/1, d²2/2  "d"
  Memory10/1 -> [v_abc]
  Gain4/1 -> abc to dq1/1
  [p_des] -> p_des/1
  Power Controllers1/2(p_des) -> [p_des]
  PLL/2(v_dq0) -> [v_dq0]
  PLL/4(x_pll) -> [x_pll]
  q²4/1 -> Sum2/2
  Current Loop/3(x_iq) -> [x_iq]
  Power Controllers1/3(q_des) -> [q_des]
  [V] -> Power Controllers1/6(|V|)
  [Pset] -> Power Controllers1/5(P_set)
  [P_abc] -> Power Controllers1/4(P_abc)
  [w_pll] -> Power Controllers1/3(w_pll)
  [Delta_x_c] -> Power Controllers1/2(Delta x_c)
  [Q_abc] -> Power Controllers1/1(Q_abc)
  [q_des] -> q_des/1
  [Qset] -> Converter State Deviation for DVPP with DC side1/3(Qset)
  [i_dq0] -> Converter State Deviation for DVPP with DC side1/1(i_dq0)
  [x_id] -> Converter State Deviation for DVPP with DC side1/4(x_id)
  Converter State Deviation for DVPP with DC side1/1(Delta x_c) -> [Delta_x_c]
  [Pset] -> Converter State Deviation for DVPP with DC side1/2(Pset)
  [x_iq] -> Converter State Deviation for DVPP with DC side1/5(x_iq)
  [Qset] -> Power Controllers1/7(Q_set)
  theta1_p/1 -> [theta1_p]
  theta1_q/1 -> [theta1_q]
  [theta1_p] -> Power Controllers1/8(theta1_p)
  [theta1_q] -> Power Controllers1/9(theta1_q)
  LTI System1/1 -> i_dc1/1
  Power Controllers1/1(i_star_dq0) -> Reference current limitation/1(i_star_dq0)
  [i_star_dq01_lim] -> Current Loop/1(i_star_dq0)
  connections:
  Universal Bridge/RConn1 -- C_dc1/LConn1 -- i_dc1/RConn1 -- G_dc1/LConn1 -- Voltage Measurement/LConn1
  Voltage Measurement/LConn2 -- Universal Bridge/RConn2 -- C_dc1/RConn1 -- i_dc1/LConn1 -- G_dc1/RConn1
  A/RConn1 -- Three-Phase V-I Measurement/RConn1
  RL Filter Element/RConn2 -- Universal Bridge/LConn2
  B/RConn1 -- Three-Phase V-I Measurement/RConn2
  C/RConn1 -- Three-Phase V-I Measurement/RConn3
  RL Filter Element/RConn3 -- Universal Bridge/LConn3
  Three-Phase V-I Measurement/LConn2 -- RL Filter Element/LConn2
  RL Filter Element/RConn1 -- Universal Bridge/LConn1
  Three-Phase V-I Measurement/LConn1 -- RL Filter Element/LConn1
  Three-Phase V-I Measurement/LConn3 -- RL Filter Element/LConn3

== system CaseStudyII_9_Bus/BESS/Converter State Deviation ==
  i_dq0 : Inport
  x_id : Inport  Port=2
  pset : Inport  Port=3
  Constant1 : Constant  Value=xid0_DVPP_1_2_pu
  Demux2 : Demux  Outputs=3
  Gain : Gain  Gain=1/vd0_DVPP_1_2_pu
  Mux : Mux  Inputs=2
  Sum : Sum  Inputs=-+|
  Sum1 : Sum  Inputs=|+-
  Delta x_c : Outport
  wires:
  i_dq0/1 -> Demux2/1
  pset/1 -> Gain/1
  Sum/1 -> Mux/1
  Demux2/1 -> Sum/2
  Gain/1 -> Sum/1
  x_id/1 -> Sum1/1
  Constant1/1 -> Sum1/2
  Mux/1 -> Delta x_c/1
  Sum1/1 -> Mux/2

== system CaseStudyII_9_Bus/BESS/Current Loop ==
  i_star_dq0 : Inport
  v_dq0 : Inport  Port=2
  i_dq0 : Inport  Port=3
  w_pll : Inport  Port=4
  Demux : Demux  Outputs=2
  Demux1 : Demux  Outputs=2
  Demux2 : Demux  Outputs=2
  Gain : Gain  Gain=kp_i_pu
  Gain1 : Gain  Gain=ki_i_pu
  Gain2 : Gain  Gain=kp_i_pu
  Gain3 : Gain  Gain=ki_i_pu
  Gain4 : Gain  Gain=w_b
  Integrator1 : Integrator  InitialCondition=xid0_DVPP_1_2_pu
  Integrator2 : Integrator  InitialCondition=xiq0_DVPP_1_2_pu
  Memory2 : Memory
  Mux : Mux  Inputs=3
  Product : Product
  Product1 : Product
  Rf : Gain  Gain=r_f_DVPP_1_2
  Rf1 : Gain  Gain=r_f_DVPP_1_2
  Selector1 : Selector  InputPortWidth=3  IndexOptions=Index vector (dialog)  Indices=[1 2]  OutputSizes=1
  Selector2 : Selector  InputPortWidth=3  IndexOptions=Index vector (dialog)  Indices=[1 2]  OutputSizes=1
  Selector3 : Selector  InputPortWidth=3  IndexOptions=Index vector (dialog)  Indices=[1 2]  OutputSizes=1
  Sum : Sum  Inputs=|+-
  Sum1 : Sum
  Sum2 : Sum  Inputs=|+-+
  Sum3 : Sum  Inputs=|++
  Sum4 : Sum
  Sum5 : Sum  Inputs=+++|
  Sum6 : Sum  Inputs=-+|
  Sum7 : Sum  Inputs=++|
  vs_0* : Constant  Value=0
  w*Lf : Gain  Gain=l_f_DVPP_1_2/w_b
  w*Lf1 : Gain  Gain=l_f_DVPP_1_2/w_b
  v_s_ref_dq0 : Outport  VectorParamsAs1DForOutWhenUnconnected=off
  x_id : Outport  Port=2  VectorParamsAs1DForOutWhenUnconnected=off
  wires:
  vs_0*/1 -> Mux/3
  Selector3/1 -> Demux2/1
  i_dq0/1 -> Selector2/1
  Selector2/1 -> Demux1/1
  Mux/1 -> v_s_ref_dq0/1
  Sum2/1 -> Sum3/1
  v_dq0/1 -> Selector3/1
  i_star_dq0/1 -> Selector1/1
  w*Lf/1 -> Sum2/2
  Sum7/1 -> Mux/2  "vs_q*"
  Sum3/1 -> Mux/1  "vs_d*"
  Sum5/1 -> Sum7/2
  Rf/1 -> Sum2/3
  Rf1/1 -> Sum5/3
  Sum/1 -> Integrator1/1, Gain/1
  Sum1/1 -> Sum2/1
  Selector1/1 -> Demux/1
  Demux/2 -> Sum6/2
  Demux/1 -> Sum/1
  w*Lf1/1 -> Sum5/1
  Demux2/1 -> Sum3/2
  Demux2/2 -> Sum7/1
  Demux1/1 -> Product/1, Rf/1, Sum/2
  Demux1/2 -> Product1/1, Rf1/1, Sum6/1
  Gain/1 -> Sum1/1
  Gain1/1 -> Sum1/2
  Gain2/1 -> Sum4/1
  Sum6/1 -> Integrator2/1, Gain2/1
  Sum4/1 -> Sum5/2
  Gain3/1 -> Sum4/2
  Integrator2/1 -> Gain3/1
  Integrator1/1 -> Memory2/1, Gain1/1
  w_pll/1 -> Gain4/1
  Product/1 -> w*Lf1/1
  Product1/1 -> w*Lf/1
  Gain4/1 -> Product1/2, Product/2
  Memory2/1 -> x_id/1

== system CaseStudyII_9_Bus/BESS/PLL ==
  v_abc : Inport
  Display : Display
  Gain : Gain  Gain=1/fb
  Integrator3 : Integrator  InitialCondition=xpll0_pu
  Selector : Selector  InputPortWidth=3  IndexOptions=Index vector (dialog)  Indices=2  OutputSizes=1
  Subsystem : Subsystem
  abc to dq0 : powerlib_meascontrol/Transformations/abc to dq0  Alignment=90 degrees behind phase A axis
  theta_pll : Outport  VectorParamsAs1DForOutWhenUnconnected=off
  v_dq0 : Outport  Port=2  VectorParamsAs1DForOutWhenUnconnected=off
  w_pll : Outport  Port=3  VectorParamsAs1DForOutWhenUnconnected=off
  x_pll : Outport  Port=4  VectorParamsAs1DForOutWhenUnconnected=off
  wires:
  Gain/1 -> w_pll/1
  Integrator3/1 -> x_pll/1
  v_abc/1 -> Subsystem/1(Vabc), abc to dq0/1
  abc to dq0/1 -> Selector/1, v_dq0/1
  Subsystem/1(Freq) -> Display/1, Gain/1
  Subsystem/2(wt) -> abc to dq0/2, theta_pll/1
  Selector/1 -> Integrator3/1

== system CaseStudyII_9_Bus/BESS/Power Controllers ==
  Q_abc : Inport
  P_abc : Inport  Port=2
  Q_set : Inport  Port=3
  Delta x_c : Inport  Port=4
  w_pll : Inport  Port=5
  P_set : Inport  Port=6
  0 : Constant  Value=0
  DVPP State Feedback Controller for Active Power Control : Subsystem
  Mux : Mux  Inputs=3
  Reactive Power Controller PI-droop control : Subsystem
  i_star_dq0 : Outport
  p_des : Outport  Port=2
  wires:
  Mux/1 -> i_star_dq0/1
  0/1 -> Mux/3
  DVPP State Feedback Controller for Active Power Control/1(p_des) -> p_des/1
  w_pll/1 -> DVPP State Feedback Controller for Active Power Control/3(w_pll)
  P_abc/1 -> DVPP State Feedback Controller for Active Power Control/1(P_abc)
  Reactive Power Controller PI-droop control/1(i_star_q) -> Mux/2
  Q_abc/1 -> Reactive Power Controller PI-droop control/1(Q_abc)
  Q_set/1 -> Reactive Power Controller PI-droop control/2(Qset)
  Delta x_c/1 -> DVPP State Feedback Controller for Active Power Control/2(Delta_x_c)
  DVPP State Feedback Controller for Active Power Control/2(i_star_d) -> Mux/1
  P_set/1 -> DVPP State Feedback Controller for Active Power Control/4(Pset)

== system CaseStudyII_9_Bus/BESS/Reference current limitation ==
  i_star_dq0 : Inport
  i_star_max : Inport  Port=2
  Demux1 : Demux  Outputs=3
  Demux2 : Demux  Outputs=3
  Divide : Product  Inputs=*/
  Minus : Sum  Inputs=+-
  Minus1 : Sum  Inputs=+++
  Minus4 : Sum  Inputs=+++
  Product{,1..4,6..7} (7 alike) : Product  RndMeth=Zero
  Saturation1 : Saturate  UpperLimit=inf  LowerLimit=0
  Sign : Signum
  Sqrt1 : Sqrt  SaturateOnIntegerOverflow=on
  Sqrt2 : Sqrt  SaturateOnIntegerOverflow=on
  Switch1 : Switch  Threshold=1
  i_star_dq0_lim : Outport  VectorParamsAs1DForOutWhenUnconnected=off
  ||i_star_dq0|| : Outport  Port=2  VectorParamsAs1DForOutWhenUnconnected=off
  ||i_star_dq0_lim|| : Outport  Port=3  VectorParamsAs1DForOutWhenUnconnected=off
  wires:
  Sqrt2/1 -> ||i_star_dq0_lim||/1
  Minus1/1 -> Sqrt2/1
  Demux2/2 -> Product3/2, Product3/1
  Product3/1 -> Minus1/2
  Demux2/1 -> Product2/1, Product2/2
  Product4/1 -> Minus1/3
  Demux2/3 -> Product4/2, Product4/1
  Product2/1 -> Minus1/1
  i_star_max/1 -> Product6/2, Minus/2
  i_star_dq0/1 -> Switch1/3, Demux1/1, Divide/1
  Switch1/1 -> i_star_dq0_lim/1, Demux2/1
  Demux1/3 -> Product7/2, Product7/1
  Product7/1 -> Minus4/3
  Product6/1 -> Switch1/1
  Divide/1 -> Product6/1
  Sign/1 -> Switch1/2
  Saturation1/1 -> Sign/1
  Demux1/2 -> Product1/2, Product1/1
  Product/1 -> Minus4/1
  Product1/1 -> Minus4/2
  Demux1/1 -> Product/1, Product/2
  Minus4/1 -> Sqrt1/1
  Sqrt1/1 -> Minus/1, ||i_star_dq0||/1, Divide/2
  Minus/1 -> Saturation1/1

== system CaseStudyII_9_Bus/PV/Converter State Deviation for DVPP with DC side ==
  i_dq0 : Inport
  Pset : Inport  Port=2
  Qset : Inport  Port=3
  x_id : Inport  Port=4
  x_iq : Inport  Port=5
  Demux2 : Demux  Outputs=3
  Gain : Gain  Gain=1/vd0_DVPP_3_2_pu
  Gain1 : Gain  Gain=-1/vd0_DVPP_3_2_pu
  Mux : Mux
  Sum1 : Sum  Inputs=+-
  Sum2 : Sum  Inputs=-+
  Sum3 : Sum  Inputs=+-
  Sum4 : Sum  Inputs=+-
  x_id_2_pu : Constant  Value=xid0_DVPP_3_2_pu
  x_iq_2_pu : Constant  Value=xiq0_DVPP_3_2_pu
  Delta x_c : Outport
  wires:
  i_dq0/1 -> Demux2/1
  Demux2/1 -> Sum2/2
  Demux2/2 -> Sum1/1
  Sum2/1 -> Mux/1
  Sum1/1 -> Mux/2
  Gain1/1 -> Sum1/2
  Pset/1 -> Gain/1
  Gain/1 -> Sum2/1
  Qset/1 -> Gain1/1
  x_id/1 -> Sum3/1
  Sum3/1 -> Mux/3
  x_id_2_pu/1 -> Sum3/2
  Mux/1 -> Delta x_c/1
  Sum4/1 -> Mux/4
  x_iq_2_pu/1 -> Sum4/2
  x_iq/1 -> Sum4/1

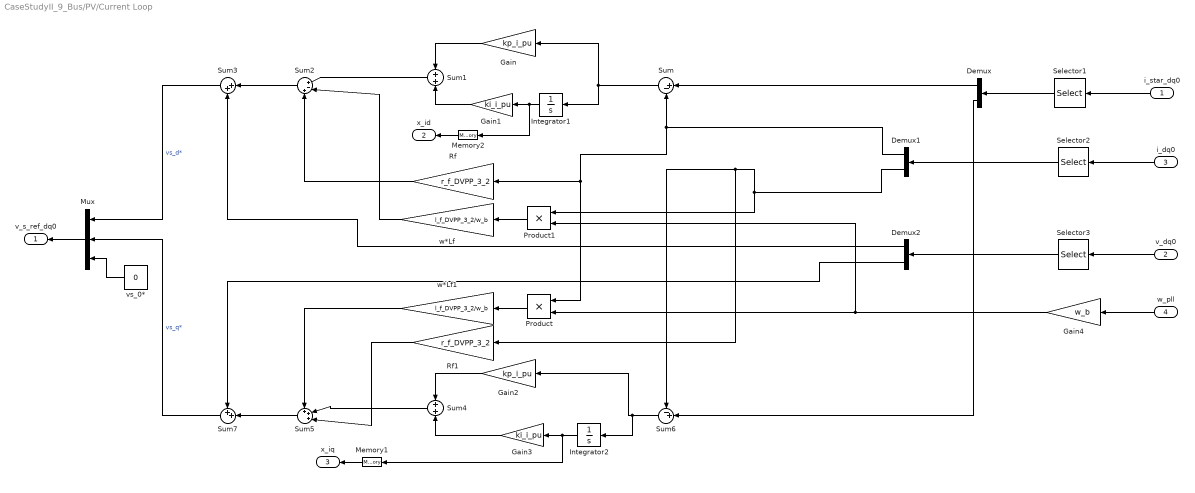
== system CaseStudyII_9_Bus/PV/Current Loop ==
  i_star_dq0 : Inport
  v_dq0 : Inport  Port=2
  i_dq0 : Inport  Port=3
  w_pll : Inport  Port=4
  Demux : Demux  Outputs=2
  Demux1 : Demux  Outputs=2
  Demux2 : Demux  Outputs=2
  Gain : Gain  Gain=kp_i_pu
  Gain1 : Gain  Gain=ki_i_pu
  Gain2 : Gain  Gain=kp_i_pu
  Gain3 : Gain  Gain=ki_i_pu
  Gain4 : Gain  Gain=w_b
  Integrator1 : Integrator  InitialCondition=xid0_DVPP_3_2_pu
  Integrator2 : Integrator  InitialCondition=xiq0_DVPP_3_2_pu
  Memory1 : Memory
  Memory2 : Memory
  Mux : Mux  Inputs=3
  Product : Product
  Product1 : Product
  Rf : Gain  Gain=r_f_DVPP_3_2
  Rf1 : Gain  Gain=r_f_DVPP_3_2
  Selector1 : Selector  InputPortWidth=3  IndexOptions=Index vector (dialog)  Indices=[1 2]  OutputSizes=1
  Selector2 : Selector  InputPortWidth=3  IndexOptions=Index vector (dialog)  Indices=[1 2]  OutputSizes=1
  Selector3 : Selector  InputPortWidth=3  IndexOptions=Index vector (dialog)  Indices=[1 2]  OutputSizes=1
  Sum : Sum  Inputs=|+-
  Sum1 : Sum
  Sum2 : Sum  Inputs=|+-+
  Sum3 : Sum  Inputs=|++
  Sum4 : Sum
  Sum5 : Sum  Inputs=+++|
  Sum6 : Sum  Inputs=-+|
  Sum7 : Sum  Inputs=++|
  vs_0* : Constant  Value=0
  w*Lf : Gain  Gain=l_f_DVPP_3_2/w_b
  w*Lf1 : Gain  Gain=l_f_DVPP_3_2/w_b
  v_s_ref_dq0 : Outport  VectorParamsAs1DForOutWhenUnconnected=off
  x_id : Outport  Port=2  VectorParamsAs1DForOutWhenUnconnected=off
  x_iq : Outport  Port=3  VectorParamsAs1DForOutWhenUnconnected=off
  wires:
  vs_0*/1 -> Mux/3
  Selector3/1 -> Demux2/1
  i_dq0/1 -> Selector2/1
  Selector2/1 -> Demux1/1
  Mux/1 -> v_s_ref_dq0/1
  Sum2/1 -> Sum3/1
  v_dq0/1 -> Selector3/1
  i_star_dq0/1 -> Selector1/1
  w*Lf/1 -> Sum2/2
  Sum7/1 -> Mux/2  "vs_q*"
  Sum3/1 -> Mux/1  "vs_d*"
  Sum5/1 -> Sum7/2
  Rf/1 -> Sum2/3
  Rf1/1 -> Sum5/3
  Sum/1 -> Integrator1/1, Gain/1
  Sum1/1 -> Sum2/1
  Selector1/1 -> Demux/1
  Demux/2 -> Sum6/2
  Demux/1 -> Sum/1
  w*Lf1/1 -> Sum5/1
  Demux2/1 -> Sum3/2
  Demux2/2 -> Sum7/1
  Demux1/1 -> Product/1, Rf/1, Sum/2
  Demux1/2 -> Product1/1, Rf1/1, Sum6/1
  Gain/1 -> Sum1/1
  Gain1/1 -> Sum1/2
  Gain2/1 -> Sum4/1
  Sum6/1 -> Integrator2/1, Gain2/1
  Sum4/1 -> Sum5/2
  Gain3/1 -> Sum4/2
  Integrator2/1 -> Memory1/1, Gain3/1
  Integrator1/1 -> Memory2/1, Gain1/1
  w_pll/1 -> Gain4/1
  Product/1 -> w*Lf1/1
  Product1/1 -> w*Lf/1
  Gain4/1 -> Product1/2, Product/2
  Memory2/1 -> x_id/1
  Memory1/1 -> x_iq/1

== system CaseStudyII_9_Bus/PV/PLL ==
  v_abc : Inport
  Display : Display
  Gain : Gain  Gain=1/fb
  Integrator3 : Integrator  InitialCondition=xpll0_pu
  Selector : Selector  InputPortWidth=3  IndexOptions=Index vector (dialog)  Indices=2  OutputSizes=1
  Subsystem : Subsystem
  abc to dq0 : powerlib_meascontrol/Transformations/abc to dq0  Alignment=90 degrees behind phase A axis
  theta_pll : Outport  VectorParamsAs1DForOutWhenUnconnected=off
  v_dq0 : Outport  Port=2  VectorParamsAs1DForOutWhenUnconnected=off
  w_pll : Outport  Port=3  VectorParamsAs1DForOutWhenUnconnected=off
  x_pll : Outport  Port=4  VectorParamsAs1DForOutWhenUnconnected=off
  wires:
  Gain/1 -> w_pll/1
  Integrator3/1 -> x_pll/1
  v_abc/1 -> Subsystem/1(Vabc), abc to dq0/1
  abc to dq0/1 -> Selector/1, v_dq0/1
  Subsystem/1(Freq) -> Display/1, Gain/1
  Subsystem/2(wt) -> abc to dq0/2, theta_pll/1
  Selector/1 -> Integrator3/1

== system CaseStudyII_9_Bus/PV/Power Controllers ==
  Q_abc : Inport
  Delta x_c : Inport  Port=2
  w_pll : Inport  Port=3
  P_abc : Inport  Port=4
  P_set : Inport  Port=5
  |V| : Inport  Port=6
  Q_set : Inport  Port=7
  theta2_p : Inport  Port=8
  theta2_q : Inport  Port=9
  0 : Constant  Value=0
  DVPP State Feedback Controller : Subsystem
  Mux : Mux  Inputs=3
  i_star_dq0 : Outport
  p_des : Outport  Port=2
  q_des : Outport  Port=3
  wires:
  0/1 -> Mux/3
  DVPP State Feedback Controller/1(i_star_d) -> Mux/1
  DVPP State Feedback Controller/3(p_des) -> p_des/1
  Q_abc/1 -> DVPP State Feedback Controller/5(Q_abc)
  |V|/1 -> DVPP State Feedback Controller/2("|V| ")
  DVPP State Feedback Controller/2(i_star_q) -> Mux/2
  DVPP State Feedback Controller/4(q_des) -> q_des/1
  w_pll/1 -> DVPP State Feedback Controller/1(w_pll)
  P_abc/1 -> DVPP State Feedback Controller/3(P_abc)
  P_set/1 -> DVPP State Feedback Controller/4(P_set)
  Delta x_c/1 -> DVPP State Feedback Controller/6(Delta_x_c)
  Mux/1 -> i_star_dq0/1
  Q_set/1 -> DVPP State Feedback Controller/7(Q_set)
  theta2_q/1 -> DVPP State Feedback Controller/9(theta2_q)
  theta2_p/1 -> DVPP State Feedback Controller/8(theta2_p)

== system CaseStudyII_9_Bus/PV/Reference current limitation ==
  i_star_dq0 : Inport
  i_star_max : Inport  Port=2
  Demux1 : Demux  Outputs=3
  Demux2 : Demux  Outputs=3
  Divide : Product  Inputs=*/
  Minus : Sum  Inputs=+-
  Minus1 : Sum  Inputs=+++
  Minus4 : Sum  Inputs=+++
  Product{,1..4,6..7} (7 alike) : Product  RndMeth=Zero
  Saturation1 : Saturate  UpperLimit=inf  LowerLimit=0
  Sign : Signum
  Sqrt1 : Sqrt  SaturateOnIntegerOverflow=on
  Sqrt2 : Sqrt  SaturateOnIntegerOverflow=on
  Switch1 : Switch  Threshold=1
  i_star_dq0_lim : Outport  VectorParamsAs1DForOutWhenUnconnected=off
  ||i_star_dq0|| : Outport  Port=2  VectorParamsAs1DForOutWhenUnconnected=off
  ||i_star_dq0_lim|| : Outport  Port=3  VectorParamsAs1DForOutWhenUnconnected=off
  wires:
  Sqrt2/1 -> ||i_star_dq0_lim||/1
  Minus1/1 -> Sqrt2/1
  Demux2/2 -> Product3/2, Product3/1
  Product3/1 -> Minus1/2
  Demux2/1 -> Product2/1, Product2/2
  Product4/1 -> Minus1/3
  Demux2/3 -> Product4/2, Product4/1
  Product2/1 -> Minus1/1
  i_star_max/1 -> Product6/2, Minus/2
  i_star_dq0/1 -> Switch1/3, Demux1/1, Divide/1
  Demux1/3 -> Product7/2, Product7/1
  Product7/1 -> Minus4/3
  Product6/1 -> Switch1/1
  Divide/1 -> Product6/1
  Sign/1 -> Switch1/2
  Saturation1/1 -> Sign/1
  Demux1/2 -> Product1/2, Product1/1
  Product/1 -> Minus4/1
  Product1/1 -> Minus4/2
  Demux1/1 -> Product/1, Product/2
  Minus4/1 -> Sqrt1/1
  Sqrt1/1 -> Minus/1, ||i_star_dq0||/1, Divide/2
  Minus/1 -> Saturation1/1
  Switch1/1 -> Demux2/1, i_star_dq0_lim/1

== system CaseStudyII_9_Bus/STATCOM with Battery/Converter State Deviation for DVPP with DC side ==
  i_dq0 : Inport
  Pset : Inport  Port=2
  Qset : Inport  Port=3
  x_id : Inport  Port=4
  x_iq : Inport  Port=5
  Demux2 : Demux  Outputs=3
  Gain : Gain  Gain=1/vd0_DVPP_3_3_pu
  Gain1 : Gain  Gain=-1/vd0_DVPP_3_3_pu
  Mux : Mux
  Sum1 : Sum  Inputs=+-
  Sum2 : Sum  Inputs=-+
  Sum3 : Sum  Inputs=+-
  Sum4 : Sum  Inputs=+-
  x_id_3_pu : Constant  Value=xid0_DVPP_3_3_pu
  x_iq_3_pu : Constant  Value=xiq0_DVPP_3_3_pu
  Delta x_c : Outport
  wires:
  i_dq0/1 -> Demux2/1
  Demux2/1 -> Sum2/2
  Demux2/2 -> Sum1/1
  Sum2/1 -> Mux/1
  Sum1/1 -> Mux/2
  Gain1/1 -> Sum1/2
  Pset/1 -> Gain/1
  Gain/1 -> Sum2/1
  Qset/1 -> Gain1/1
  x_id/1 -> Sum3/1
  Sum3/1 -> Mux/3
  x_id_3_pu/1 -> Sum3/2
  Mux/1 -> Delta x_c/1
  Sum4/1 -> Mux/4
  x_iq_3_pu/1 -> Sum4/2
  x_iq/1 -> Sum4/1

== system CaseStudyII_9_Bus/STATCOM with Battery/Current Loop ==
  i_star_dq0 : Inport
  v_dq0 : Inport  Port=2
  i_dq0 : Inport  Port=3
  w_pll : Inport  Port=4
  Demux : Demux  Outputs=2
  Demux1 : Demux  Outputs=2
  Demux2 : Demux  Outputs=2
  Gain : Gain  Gain=kp_i_pu
  Gain1 : Gain  Gain=ki_i_pu
  Gain2 : Gain  Gain=kp_i_pu
  Gain3 : Gain  Gain=ki_i_pu
  Gain4 : Gain  Gain=w_b
  Integrator1 : Integrator  InitialCondition=xid0_DVPP_3_3_pu
  Integrator2 : Integrator  InitialCondition=xiq0_DVPP_3_3_pu
  Memory1 : Memory
  Memory2 : Memory
  Mux : Mux  Inputs=3
  Product : Product
  Product1 : Product
  Rf : Gain  Gain=r_f_DVPP_3_3
  Rf1 : Gain  Gain=r_f_DVPP_3_3
  Selector1 : Selector  InputPortWidth=3  IndexOptions=Index vector (dialog)  Indices=[1 2]  OutputSizes=1
  Selector2 : Selector  InputPortWidth=3  IndexOptions=Index vector (dialog)  Indices=[1 2]  OutputSizes=1
  Selector3 : Selector  InputPortWidth=3  IndexOptions=Index vector (dialog)  Indices=[1 2]  OutputSizes=1
  Sum : Sum  Inputs=|+-
  Sum1 : Sum
  Sum2 : Sum  Inputs=|+-+
  Sum3 : Sum  Inputs=|++
  Sum4 : Sum
  Sum5 : Sum  Inputs=+++|
  Sum6 : Sum  Inputs=-+|
  Sum7 : Sum  Inputs=++|
  vs_0* : Constant  Value=0
  w*Lf : Gain  Gain=l_f_DVPP_3_3/w_b
  w*Lf1 : Gain  Gain=l_f_DVPP_3_3/w_b
  v_s_ref_dq0 : Outport  VectorParamsAs1DForOutWhenUnconnected=off
  x_id : Outport  Port=2  VectorParamsAs1DForOutWhenUnconnected=off
  x_iq : Outport  Port=3  VectorParamsAs1DForOutWhenUnconnected=off
  wires:
  vs_0*/1 -> Mux/3
  Selector3/1 -> Demux2/1
  i_dq0/1 -> Selector2/1
  Selector2/1 -> Demux1/1
  Mux/1 -> v_s_ref_dq0/1
  Sum2/1 -> Sum3/1
  v_dq0/1 -> Selector3/1
  i_star_dq0/1 -> Selector1/1
  w*Lf/1 -> Sum2/2
  Sum7/1 -> Mux/2  "vs_q*"
  Sum3/1 -> Mux/1  "vs_d*"
  Sum5/1 -> Sum7/2
  Rf/1 -> Sum2/3
  Rf1/1 -> Sum5/3
  Sum/1 -> Integrator1/1, Gain/1
  Sum1/1 -> Sum2/1
  Selector1/1 -> Demux/1
  Demux/2 -> Sum6/2
  Demux/1 -> Sum/1
  w*Lf1/1 -> Sum5/1
  Demux2/1 -> Sum3/2
  Demux2/2 -> Sum7/1
  Demux1/1 -> Product/1, Rf/1, Sum/2
  Demux1/2 -> Product1/1, Rf1/1, Sum6/1
  Gain/1 -> Sum1/1
  Gain1/1 -> Sum1/2
  Gain2/1 -> Sum4/1
  Sum6/1 -> Integrator2/1, Gain2/1
  Sum4/1 -> Sum5/2
  Gain3/1 -> Sum4/2
  Integrator2/1 -> Memory1/1, Gain3/1
  Integrator1/1 -> Memory2/1, Gain1/1
  w_pll/1 -> Gain4/1
  Product/1 -> w*Lf1/1
  Product1/1 -> w*Lf/1
  Gain4/1 -> Product1/2, Product/2
  Memory2/1 -> x_id/1
  Memory1/1 -> x_iq/1

== system CaseStudyII_9_Bus/STATCOM with Battery/PLL ==
  v_abc : Inport
  Display : Display
  Gain : Gain  Gain=1/fb
  Integrator3 : Integrator  InitialCondition=xpll0_pu
  Selector : Selector  InputPortWidth=3  IndexOptions=Index vector (dialog)  Indices=2  OutputSizes=1
  Subsystem : Subsystem
  abc to dq0 : powerlib_meascontrol/Transformations/abc to dq0  Alignment=90 degrees behind phase A axis
  theta_pll : Outport  VectorParamsAs1DForOutWhenUnconnected=off
  v_dq0 : Outport  Port=2  VectorParamsAs1DForOutWhenUnconnected=off
  w_pll : Outport  Port=3  VectorParamsAs1DForOutWhenUnconnected=off
  x_pll : Outport  Port=4  VectorParamsAs1DForOutWhenUnconnected=off
  wires:
  Gain/1 -> w_pll/1
  Integrator3/1 -> x_pll/1
  v_abc/1 -> Subsystem/1(Vabc), abc to dq0/1
  abc to dq0/1 -> Selector/1, v_dq0/1
  Subsystem/1(Freq) -> Display/1, Gain/1
  Subsystem/2(wt) -> abc to dq0/2, theta_pll/1
  Selector/1 -> Integrator3/1
